simulink model "Model_with_RL_only"  (R2020b)
settings: Solver=VariableStepAuto  StartTime=0.0  StopTime=10  FixedStep=0.00001  RelTol=1e-3
values from neighbouring files (symbols this model uses):
  b = 0.0001    [RL_model_parameters.m]
  basel = 0.332    [RL_model_parameters.m]
  Izz = 0.8    [RL_model_parameters.m]
  Kb = 0.031    [RL_model_parameters.m]
  Kt = 0.016    [RL_model_parameters.m]
  L = 0.05    [RL_model_parameters.m]
  m = 40    [RL_model_parameters.m]
  NN = 1    [RL_model_parameters.m]
  r = 0.06    [RL_model_parameters.m]
  RR = 1    [RL_model_parameters.m]
settings Model: Creator=FUJITSU  LastModifiedBy=mohamed mohssen
settings SolverCC: ConsecutiveZCsStepRelTol=1e-4

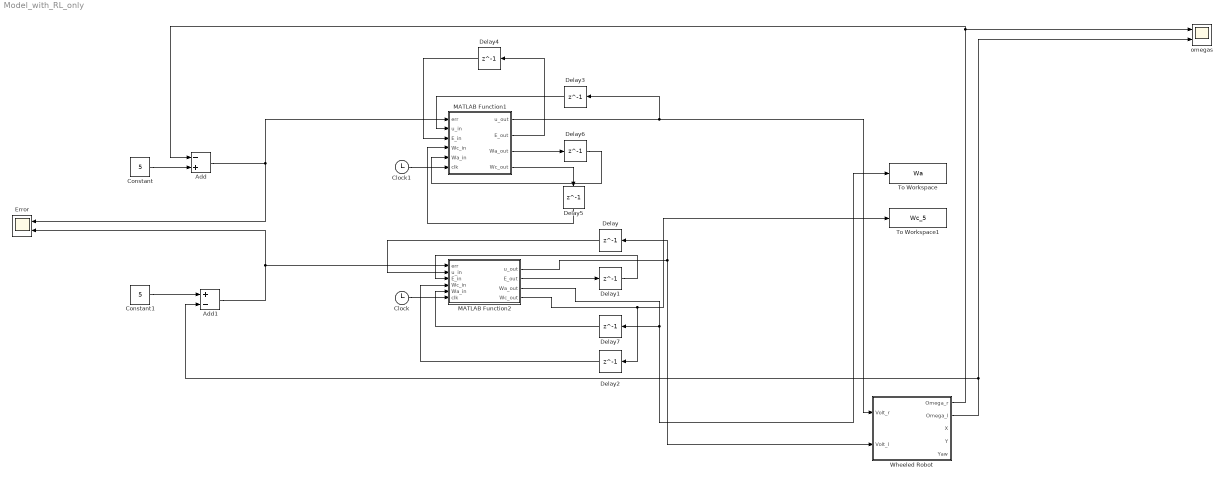
== system Model_with_RL_only ==
  Add : Sum  Inputs=-+
  Add1 : Sum  Inputs=+-
  Clock : Clock
  Clock1 : Clock
  Constant : Constant  Value=5  SampleTime=0.01
  Constant1 : Constant  Value=5  SampleTime=0.01
  Delay : Delay  DelayLength=1  InitialCondition=0  SampleTime=0.01
  Delay{1,4,6..7} (4 alike) : Delay  DelayLength=1  InitialCondition=[0;0;0]  SampleTime=0.01
  Delay2 : Delay  DelayLength=1  InitialCondition=[0,0,0,0;0,0,0,0;0,0,0,0;0,0,0,0]  SampleTime=0.01
  Delay3 : Delay  DelayLength=1  InitialCondition=0  SampleTime=0.01
  Delay5 : Delay  DelayLength=1  InitialCondition=[0,0,0,0;0,0,0,0;0,0,0,0;0,0,0,0]  SampleTime=0.01
  Error : Scope  NumInputPorts=2
  MATLAB Function1 : MATLAB Function  TreatAsAtomicUnit=on
  MATLAB Function2 : MATLAB Function  TreatAsAtomicUnit=on
  To Workspace : ToWorkspace  VariableName=Wa  SampleTime=0.01
  To Workspace1 : ToWorkspace  VariableName=Wc_5  SampleTime=0.01
  Wheeled Robot : Subsystem
  omegas : Scope  NumInputPorts=2
  wires:
  Wheeled Robot/1(Omega_r) -> Add/1, omegas/1
  Wheeled Robot/2(Omega_l) -> omegas/2, Add1/2
  MATLAB Function2/2(E_out) -> Delay1/1
  Clock1/1 -> MATLAB Function1/6(clk)
  MATLAB Function1/2(E_out) -> Delay4/1
  Delay4/1 -> MATLAB Function1/3(E_in)
  Add/1 -> Error/1, MATLAB Function1/1(err)
  Add1/1 -> Error/2, MATLAB Function2/1(err)
  MATLAB Function1/4(Wc_out) -> Delay5/1
  MATLAB Function1/3(Wa_out) -> Delay6/1
  Delay6/1 -> MATLAB Function1/5(Wa_in)
  Delay5/1 -> MATLAB Function1/4(Wc_in)
  Delay1/1 -> MATLAB Function2/3(E_in)
  MATLAB Function2/4(Wc_out) -> To Workspace1/1, Delay2/1
  Delay2/1 -> MATLAB Function2/4(Wc_in)
  MATLAB Function2/3(Wa_out) -> To Workspace/1, Delay7/1
  Delay7/1 -> MATLAB Function2/5(Wa_in)
  Clock/1 -> MATLAB Function2/6(clk)
  Delay3/1 -> MATLAB Function1/2(u_in)
  Delay/1 -> MATLAB Function2/2(u_in)
  MATLAB Function1/1(u_out) -> Wheeled Robot/1(Volt_r), Delay3/1
  MATLAB Function2/1(u_out) -> Wheeled Robot/2(Volt_l), Delay/1
  Constant/1 -> Add/2
  Constant1/1 -> Add1/1

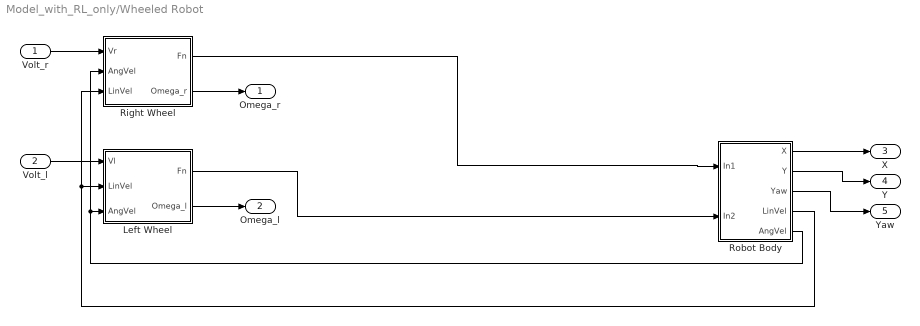
== system Model_with_RL_only/Wheeled Robot ==
  Volt_r : Inport
  Volt_l : Inport  Port=2
  Left Wheel : Subsystem
  Right Wheel : Subsystem
  Robot Body : Subsystem
  Omega_r : Outport
  Omega_l : Outport  Port=2
  X : Outport  Port=3
  Y : Outport  Port=4
  Yaw : Outport  Port=5
  wires:
  Robot Body/1(X) -> X/1
  Robot Body/3(Yaw) -> Yaw/1
  Right Wheel/1(Fn) -> Robot Body/1(In1)
  Volt_r/1 -> Right Wheel/1(Vr)
  Volt_l/1 -> Left Wheel/1(Vl)
  Left Wheel/2(Omega_l) -> Omega_l/1
  Robot Body/2(Y) -> Y/1
  Robot Body/4(LinVel) -> Left Wheel/2(LinVel), Right Wheel/3(LinVel)
  Robot Body/5(AngVel) -> Left Wheel/3(AngVel), Right Wheel/2(AngVel)
  Left Wheel/1(Fn) -> Robot Body/2(In2)
  Right Wheel/2(Omega_r) -> Omega_r/1

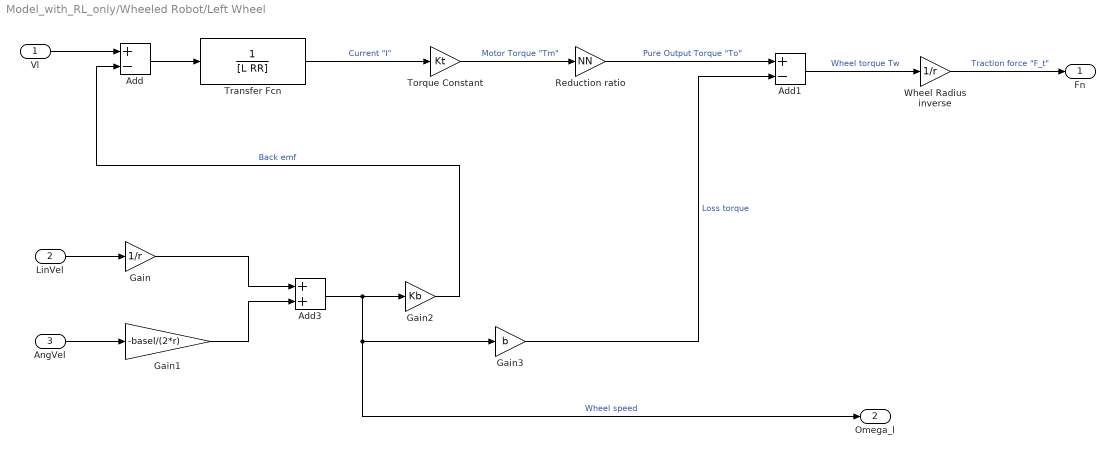
== system Model_with_RL_only/Wheeled Robot/Left Wheel ==
  Vl : Inport
  LinVel : Inport  Port=2
  AngVel : Inport  Port=3
  Add : Sum  Inputs=+-
  Add1 : Sum  Inputs=+-
  Add3 : Sum
  Gain : Gain  Gain=1/r
  Gain1 : Gain  Gain=-basel/(2*r)
  Gain2 : Gain  Gain=Kb
  Gain3 : Gain  Gain=b
  Reduction ratio : Gain  Gain=NN
  Torque Constant : Gain  Gain=Kt
  Transfer Fcn : TransferFcn  Denominator=[L RR]  AbsoluteTolerance=0.01
  Wheel Radius inverse : Gain  Gain=1/r
  Fn : Outport
  Omega_l : Outport  Port=2
  wires:
  Wheel Radius inverse/1 -> Fn/1  "Traction force \"F_t\""
  Add/1 -> Transfer Fcn/1
  Torque Constant/1 -> Reduction ratio/1  "Motor Torque \"Tm\""
  Add1/1 -> Wheel Radius inverse/1  "Wheel torque Tw"
  Transfer Fcn/1 -> Torque Constant/1  "Current \"I\""
  Reduction ratio/1 -> Add1/1  "Pure Output Torque \"To\""
  Vl/1 -> Add/1
  Gain1/1 -> Add3/2
  AngVel/1 -> Gain1/1
  Add3/1 -> Gain3/1, Omega_l/1, Gain2/1  "Wheel speed"
  Gain2/1 -> Add/2  "Back emf"
  Gain3/1 -> Add1/2  "Loss torque"
  Gain/1 -> Add3/1
  LinVel/1 -> Gain/1

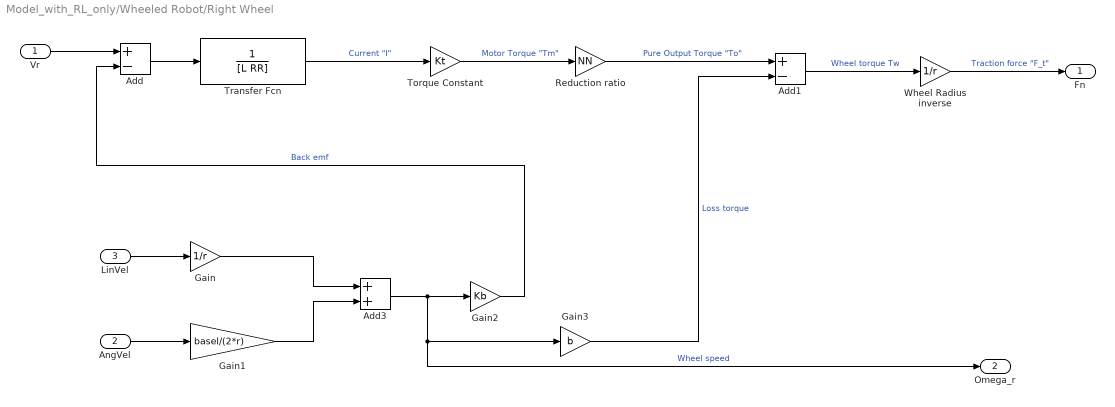
== system Model_with_RL_only/Wheeled Robot/Right Wheel ==
  Vr : Inport
  AngVel : Inport  Port=2
  LinVel : Inport  Port=3
  Add : Sum  Inputs=+-
  Add1 : Sum  Inputs=+-
  Add3 : Sum
  Gain : Gain  Gain=1/r
  Gain1 : Gain  Gain=basel/(2*r)
  Gain2 : Gain  Gain=Kb
  Gain3 : Gain  Gain=b
  Reduction ratio : Gain  Gain=NN
  Torque Constant : Gain  Gain=Kt
  Transfer Fcn : TransferFcn  Denominator=[L RR]
  Wheel Radius inverse : Gain  Gain=1/r
  Fn : Outport
  Omega_r : Outport  Port=2
  wires:
  Wheel Radius inverse/1 -> Fn/1  "Traction force \"F_t\""
  Add/1 -> Transfer Fcn/1
  Torque Constant/1 -> Reduction ratio/1  "Motor Torque \"Tm\""
  Add1/1 -> Wheel Radius inverse/1  "Wheel torque Tw"
  Transfer Fcn/1 -> Torque Constant/1  "Current \"I\""
  Reduction ratio/1 -> Add1/1  "Pure Output Torque \"To\""
  Vr/1 -> Add/1
  LinVel/1 -> Gain/1
  AngVel/1 -> Gain1/1
  Gain/1 -> Add3/1
  Gain1/1 -> Add3/2
  Add3/1 -> Gain3/1, Omega_r/1, Gain2/1  "Wheel speed"
  Gain2/1 -> Add/2  "Back emf"
  Gain3/1 -> Add1/2  "Loss torque"

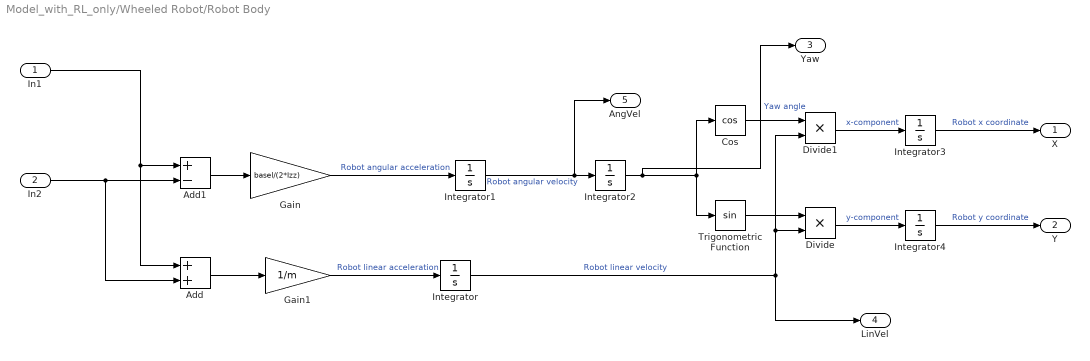
== system Model_with_RL_only/Wheeled Robot/Robot Body ==
  In1 : Inport
  In2 : Inport  Port=2
  Add : Sum
  Add1 : Sum  Inputs=+-
  Cos : Trigonometry  Operator=cos
  Divide : Product  Inputs=**
  Divide1 : Product  Inputs=**
  Gain : Gain  Gain=basel/(2*Izz)
  Gain1 : Gain  Gain=1/m
  Integrator{,1..4} (5 alike) : Integrator
  Trigonometric Function : Trigonometry
  X : Outport
  Y : Outport  Port=2
  Yaw : Outport  Port=3
  LinVel : Outport  Port=4
  AngVel : Outport  Port=5
  wires:
  Integrator3/1 -> X/1  "Robot x coordinate"
  Integrator1/1 -> AngVel/1, Integrator2/1  "Robot angular velocity"
  In2/1 -> Add1/2, Add/2
  Integrator/1 -> LinVel/1, Divide1/2, Divide/2  "Robot linear velocity"
  In1/1 -> Add/1, Add1/1
  Add/1 -> Gain1/1
  Add1/1 -> Gain/1
  Integrator2/1 -> Yaw/1, Trigonometric Function/1, Cos/1  "Yaw angle"
  Trigonometric Function/1 -> Divide/1
  Integrator4/1 -> Y/1  "Robot y coordinate"
  Divide1/1 -> Integrator3/1  "x-component"
  Gain/1 -> Integrator1/1  "Robot angular acceleration"
  Gain1/1 -> Integrator/1  "Robot linear acceleration"
  Divide/1 -> Integrator4/1  "y-component"
  Cos/1 -> Divide1/1

== matlab function Model_with_RL_only/MATLAB Function2 ==
  settings: updateMethod=DISCRETE
  data: u_out output; err input; u_in input; E_in input; Wc_in input; Wa_in input; clk input; E_out output; Wa_out output; Wc_out output
function [u_out, E_out, Wa_out,Wc_out] = RL(err, u_in, E_in, Wc_in,Wa_in, clk)
 r = 1.1 ; 
 q = 2 * eye(3); 
 
 alpha_a=0.001; alpha_c=0.001;
 if clk<=0
  
    Wc_in=[1,1,1,0.9;1,1,1,0.9;1,1,1,1;0.9,.9,1,1000];
    %Wa_in=[12.3111  ; 11.8884 ; 12.0631];
    
    Wa_in=[1200; 10; 0];
    
    e_k1 = 0 ;
    e_k2 = 0 ;
    e_k3 = 0 ;
    E_in = [e_k1 ; e_k2 ; e_k3];
    u_in = 5;
 end
    e_k1 = E_in(1) ;
    e_k3 = E_in(3);
    e_k2 = E_in(2);
    E_k = [e_k1 ; e_k2 ; e_k3];  
    u_out = (Wa_in'*E_k )+5;
    u_des= -(1/Wc_in(4,4))*(Wc_in(4,1:3)) * E_k ;
    Wa_o=Wa_in'-(alpha_a*(u_out-u_des)*E_k');
    Wa_out=Wa_o';
    e_k3 = E_in(2);
    e_k2 = E_in(1);
    e_k1 = err;
    E_k_plus_1 = [e_k1 ; e_k2 ; e_k3];
    z_k=[E_k',(u_in)]/2;
    z_k_1=[E_k_plus_1',(u_out)]/2;
    v_k=0.5*z_k*Wc_in*z_k';
    v_k_1=0.5*z_k_1*Wc_in*z_k_1';
    v_des=0.5*(E_k'*q*E_k+(1/u_out)*r*u_out)+v_k_1;
    Wc_out=Wc_in-(alpha_c*(v_k-v_des)*(z_k'*z_k));
    E_out=E_k_plus_1;

== matlab function Model_with_RL_only/MATLAB Function1 ==
  settings: updateMethod=DISCRETE
  data: u_out output; err input; u_in input; E_in input; Wc_in input; Wa_in input; clk input; E_out output; Wa_out output; Wc_out output
function [u_out, E_out, Wa_out,Wc_out] = RL(err, u_in, E_in, Wc_in,Wa_in, clk)
 r = 1.1 ; 
 q = 2 * eye(3); 
 
 alpha_a=0.001; alpha_c=0.001;
 if clk<=0
  
    Wc_in=[1,1,1,0.9;1,1,1,0.9;1,1,1,1;0.9,.9,1,1000];
    %Wa_in=[12.3111  ; 11.8884 ; 12.0631];
    
    Wa_in=[1200; 10; 0];
    
    e_k1 = 0 ;
    e_k2 = 0 ;
    e_k3 = 0 ;
    E_in = [e_k1 ; e_k2 ; e_k3];
    u_in = 5;
 end
    e_k1 = E_in(1) ;
    e_k3 = E_in(3);
    e_k2 = E_in(2);
    E_k = [e_k1 ; e_k2 ; e_k3];  
    u_out = (Wa_in'*E_k )+5;
    u_des= -(1/Wc_in(4,4))*(Wc_in(4,1:3)) * E_k ;
    Wa_o=Wa_in'-(alpha_a*(u_out-u_des)*E_k');
    Wa_out=Wa_o';
    e_k3 = E_in(2);
    e_k2 = E_in(1);
    e_k1 = err;
    E_k_plus_1 = [e_k1 ; e_k2 ; e_k3];
    z_k=[E_k',(u_in)]/2;
    z_k_1=[E_k_plus_1',(u_out)]/2;
    v_k=0.5*z_k*Wc_in*z_k';
    v_k_1=0.5*z_k_1*Wc_in*z_k_1';
    v_des=0.5*(E_k'*q*E_k+(1/u_out)*r*u_out)+v_k_1;
    Wc_out=Wc_in-(alpha_c*(v_k-v_des)*(z_k'*z_k));
    E_out=E_k_plus_1;
